simulink model "hcs_new"  (R2018a)
settings: Solver=VariableStepAuto  StartTime=0.0  StopTime=33  RelTol=1e-3
settings Model: Creator=BEAR  LastModifiedBy=BEAR

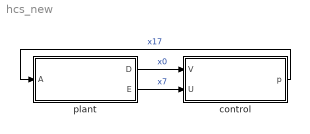
== system hcs_new ==
  control : Subsystem
  plant : Subsystem
  wires:
  control/1(p) -> plant/1(A)  "x17"
  plant/2(E) -> control/2(U)  "x7"
  plant/1(D) -> control/1(V)  "x0"

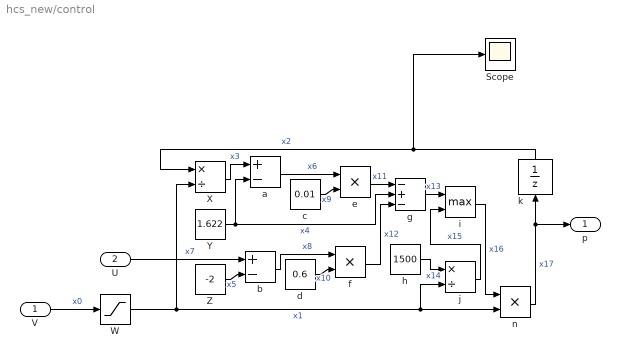
== system hcs_new/control ==
  V : Inport
  U : Inport  Port=2
  Scope : Scope
  W : Saturate  UpperLimit=800  LowerLimit=600
  X : Product  Inputs=*/  SampleTime=0.128
  Y : Constant  Value=1.622
  Z : Constant  Value=-2
  a : Sum  Inputs=+-  SampleTime=0.128
  b : Sum  Inputs=+-  SampleTime=0.128
  c : Constant  Value=0.01
  d : Constant  Value=0.6
  e : Product  Inputs=**  SampleTime=0.128
  f : Product  Inputs=**  SampleTime=0.128
  g : Sum  Inputs=-+-  SampleTime=0.128
  h : Constant  Value=1500
  i : MinMax  Function=max  Inputs=2  SampleTime=0.128
  j : Product  Inputs=*/  SampleTime=0.128
  k : UnitDelay  InitialCondition=2027.5  SampleTime=0.128
  n : Product  Inputs=**  SampleTime=0.128
  p : Outport
  wires:
  X/1 -> a/1  "x3"
  Y/1 -> g/2, a/2  "x4"
  a/1 -> e/1  "x6"
  c/1 -> e/2  "x9"
  Z/1 -> b/2  "x5"
  b/1 -> f/1  "x8"
  d/1 -> f/2  "x10"
  f/1 -> g/3  "x12"
  U/1 -> b/1  "x7"
  g/1 -> i/1  "x13"
  k/1 -> Scope/1, X/1  "x2"
  e/1 -> g/1  "x11"
  W/1 -> n/2, j/2, X/2  "x1"
  n/1 -> k/1, p/1  "x17"
  i/1 -> n/1  "x16"
  h/1 -> j/1  "x14"
  j/1 -> i/2  "x15"
  V/1 -> W/1  "x0"

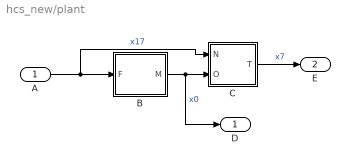
== system hcs_new/plant ==
  A : Inport
  B : Subsystem
  C : Subsystem
  D : Outport
  E : Outport  Port=2
  wires:
  B/1(M) -> C/2(O), D/1  "x0"
  C/1(T) -> E/1  "x7"
  A/1 -> C/1(N), B/1(F)  "x17"

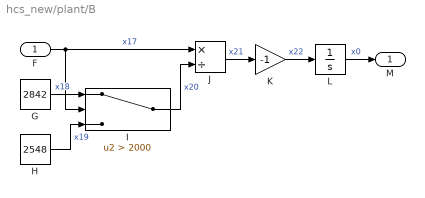
== system hcs_new/plant/B ==
  F : Inport
  G : Constant  Value=2842
  H : Constant  Value=2548
  I : Switch  Criteria=u2 > Threshold  Threshold=2000
  J : Product  Inputs=*/
  K : Gain  Gain=-1
  L : Integrator  InitialCondition=1250
  M : Outport
  wires:
  F/1 -> J/1, I/2  "x17"
  J/1 -> K/1  "x21"
  K/1 -> L/1  "x22"
  L/1 -> M/1  "x0"
  G/1 -> I/1  "x18"
  H/1 -> I/3  "x19"
  I/1 -> J/2  "x20"

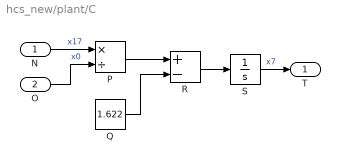
== system hcs_new/plant/C ==
  N : Inport
  O : Inport  Port=2
  P : Product  Inputs=*/
  Q : Constant  Value=1.622
  R : Sum  Inputs=+-
  S : Integrator  InitialCondition=-2
  T : Outport
  wires:
  N/1 -> P/1  "x17"
  O/1 -> P/2  "x0"
  P/1 -> R/1
  Q/1 -> R/2
  R/1 -> S/1
  S/1 -> T/1  "x7"
